simulink model "BumplessPID_UuT_Harness2"  (R2020a)
settings: Solver=ode8  StartTime=0.0  StopTime=40  FixedStep=0.1  RelTol=1e-3
libraries: SignalEditorBlockLib x1
settings Model: Creator=Christian  LastModifiedBy=Christian

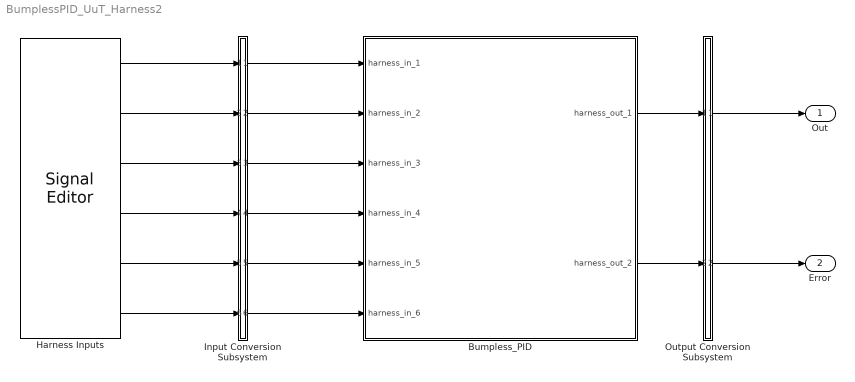
== system BumplessPID_UuT_Harness2 ==
  Bumpless_PID : Subsystem  Tag=__SL_testing_harness_stub_
  Harness Inputs : SignalEditorBlockLib/Signal Editor  FileName=ParamSweepBaseline.mat  ActiveScenario=Ki01  ActiveSignal=Bump_Rate  IsBus=off  OutputBusObjectStr=Bus: BusObject  SampleTime=0  Interpolate=off  ZeroCross=off  OutputAfterFinalValue=Setting to zero  Unit=inherit  PreserveSignalName=on
  Input Conversion Subsystem : Subsystem  Tag=__SLT_ICS__  Description=|
      | Signal spec.
      | and routing
      settings: AttributesFormatString=%<Description>
  Output Conversion Subsystem : Subsystem  Tag=__SLT_OCS__  Description=|
      | Signal spec.
      | and routing
      settings: AttributesFormatString=%<Description>
  Out : Outport
  Error : Outport  Port=2
  wires:
  Harness Inputs/1 -> Input Conversion Subsystem/1(Inport_1)
  Harness Inputs/2 -> Input Conversion Subsystem/2(Inport_2)
  Harness Inputs/3 -> Input Conversion Subsystem/3(Inport_3)
  Harness Inputs/4 -> Input Conversion Subsystem/4(Inport_4)
  Harness Inputs/5 -> Input Conversion Subsystem/5(Inport_5)
  Harness Inputs/6 -> Input Conversion Subsystem/6(Inport_6)
  Output Conversion Subsystem/1(Outport_1) -> Out/1
  Bumpless_PID/1(harness_out_1) -> Output Conversion Subsystem/1(Inport_1)
  Bumpless_PID/2(harness_out_2) -> Output Conversion Subsystem/2(Inport_2)
  Input Conversion Subsystem/1(Outport_1) -> Bumpless_PID/1(harness_in_1)
  Input Conversion Subsystem/2(Outport_2) -> Bumpless_PID/2(harness_in_2)
  Input Conversion Subsystem/3(Outport_3) -> Bumpless_PID/3(harness_in_3)
  Input Conversion Subsystem/4(Outport_4) -> Bumpless_PID/4(harness_in_4)
  Input Conversion Subsystem/5(Outport_5) -> Bumpless_PID/5(harness_in_5)
  Input Conversion Subsystem/6(Outport_6) -> Bumpless_PID/6(harness_in_6)
  Output Conversion Subsystem/2(Outport_2) -> Error/1

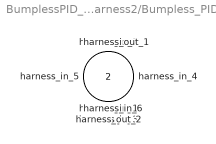
== system BumplessPID_UuT_Harness2/Bumpless_PID ==
  harness_in_1 : Inport
  harness_in_2 : Inport  Port=2
  harness_in_3 : Inport  Port=3
  harness_in_4 : Inport  Port=4
  harness_in_5 : Inport  Port=5
  harness_in_6 : Inport  Port=6
  harness_out_1 : Outport
  harness_out_2 : Outport  Port=2

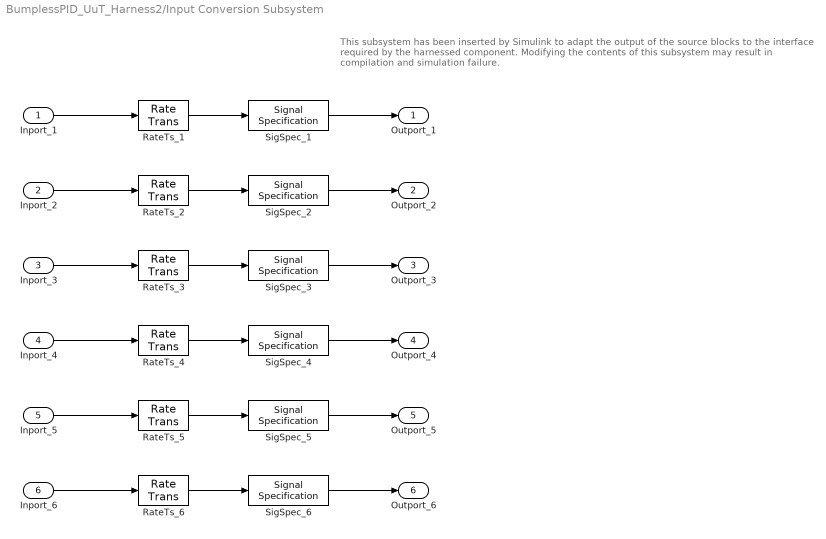
== system BumplessPID_UuT_Harness2/Input Conversion Subsystem ==
  note: This subsystem has been inserted by Simulink to adapt the output of the source blocks to the interface required by the harnessed component.
      |  Modifying the contents of this subsystem may result in compilation and simulation failure.
  Inport_1 : Inport
  Inport_2 : Inport  Port=2
  Inport_3 : Inport  Port=3
  Inport_4 : Inport  Port=4
  Inport_5 : Inport  Port=5
  Inport_6 : Inport  Port=6
  RateTs_{1..6} (6 alike) : RateTransition  OutPortSampleTime=[-1, 0]
  SigSpec_{1..6} (6 alike) : SignalSpecification  OutDataTypeStr=double  Dimensions=[1]  SampleTime=[-1, 0]
  Outport_1 : Outport
  Outport_2 : Outport  Port=2
  Outport_3 : Outport  Port=3
  Outport_4 : Outport  Port=4
  Outport_5 : Outport  Port=5
  Outport_6 : Outport  Port=6
  wires:
  SigSpec_1/1 -> Outport_1/1
  RateTs_1/1 -> SigSpec_1/1
  Inport_1/1 -> RateTs_1/1
  SigSpec_2/1 -> Outport_2/1
  RateTs_2/1 -> SigSpec_2/1
  Inport_2/1 -> RateTs_2/1
  SigSpec_3/1 -> Outport_3/1
  RateTs_3/1 -> SigSpec_3/1
  Inport_3/1 -> RateTs_3/1
  SigSpec_4/1 -> Outport_4/1
  RateTs_4/1 -> SigSpec_4/1
  Inport_4/1 -> RateTs_4/1
  SigSpec_5/1 -> Outport_5/1
  RateTs_5/1 -> SigSpec_5/1
  Inport_5/1 -> RateTs_5/1
  SigSpec_6/1 -> Outport_6/1
  RateTs_6/1 -> SigSpec_6/1
  Inport_6/1 -> RateTs_6/1

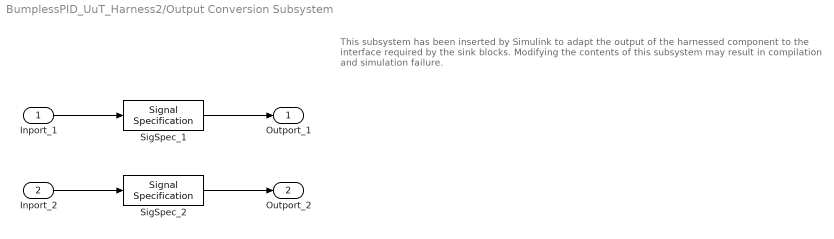
== system BumplessPID_UuT_Harness2/Output Conversion Subsystem ==
  note: This subsystem has been inserted by Simulink to adapt the output of the harnessed component to the interface required by the sink blocks.
      |  Modifying the contents of this subsystem may result in compilation and simulation failure.
  Inport_1 : Inport
  Inport_2 : Inport  Port=2
  SigSpec_1 : SignalSpecification  OutDataTypeStr=double  Dimensions=[1]
  SigSpec_2 : SignalSpecification  OutDataTypeStr=double  Dimensions=[1]  SampleTime=0.1
  Outport_1 : Outport
  Outport_2 : Outport  Port=2
  wires:
  Inport_1/1 -> SigSpec_1/1
  SigSpec_1/1 -> Outport_1/1
  Inport_2/1 -> SigSpec_2/1
  SigSpec_2/1 -> Outport_2/1
